simulink model "RF_TX_Model"  (R2026a)
settings: Solver=VariableStepAuto
InitFcn:
  | warning('off')
model workspace (MAT data in the model file):
  Az = 30
  phaseShifts = [20.1529923745; -88.4621483039; 162.922711018; 54.3075703392; -54.3075703392; -162.922711018; 88.4621483039; -20.1529923745]
values from neighbouring files (symbols this model uses):
  BW = 1e8    (= 100000000)    [MatchingNetworkDesign.m]    (also in analyzeReferenceRFBudget.m; build12GHzTransmitterRFBudget.m; build12GHzTransmitterRFBudget_Pin20dBm.m; buildReferenceRFBudgetAnalyzer.m)
  fIF = 4e9    (= 4000000000)    [analyze12GHzTransmitterBudget.m]    (also in analyzeReferenceRFBudget.m; build12GHzTransmitterRFBudget.m; build12GHzTransmitterRFBudget_Pin20dBm.m; buildReferenceRFBudgetAnalyzer.m)
  S = sparameters(rfAntenna,fRF)    [runAntenna2Bits.m]
  splitterCorporate = design(powerDividerCorporate(NumOutputPorts=N,SplitterElement=e), fRF)    [runAntenna2Bits.m]
undefined symbols (not defined in the file or in its folder): rational, sparameters
libraries: simrfV2elements x7, simrfV2_lib x6, dspstat3 x5, simrfV2util1 x3, commrflib2 x1, simrfV2systems x1, simrfV2private x1, dspmathops x1
(part 1 of 3)
settings Model: Creator=gzucchel  LastModifiedBy=gzucchel
settings DataIOCC: SaveFinalState=on  SaveOperatingPoint=on

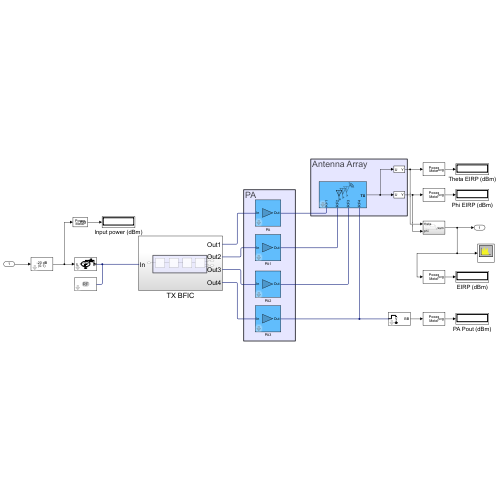
[thumbnail: Simulink's stored preview of the top-level diagram]
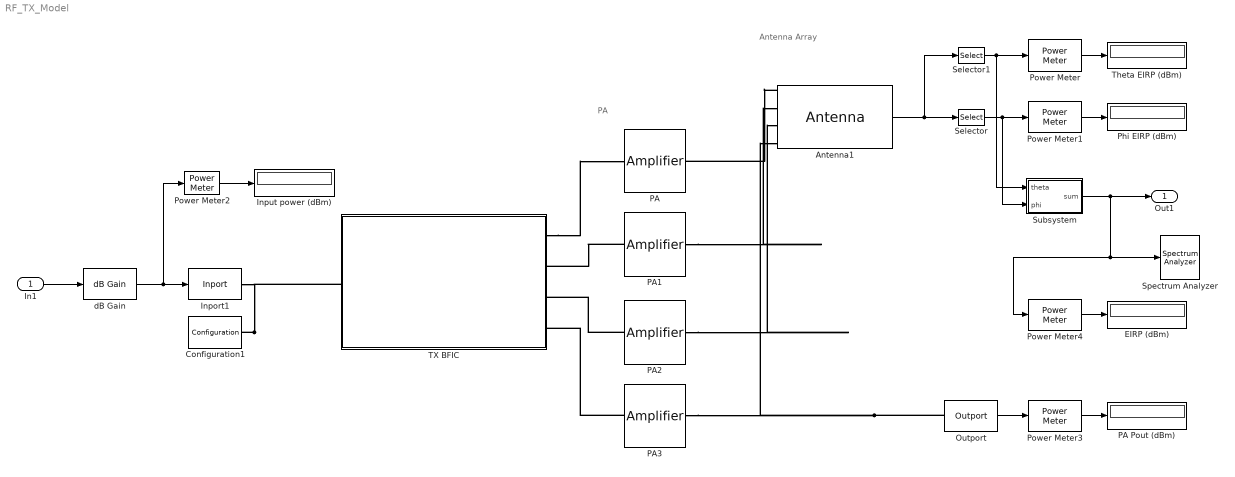
== system RF_TX_Model ==
  note: Antenna Array
  note: PA
  In1 : Inport  PortDimensions=1  SampleTime=2.03450520833333e-09  Interpolate=off
      settings: SignalType=complex
  Antenna1 : simrfV2elements/Antenna  CacheLevel=0  AntennaSource=Antenna object  PrevAppliedAntSource=Antenna object  Gr=0 dBi  Zin=50  AntennaObj=antennaArray  InputIncWave=off  OutputRadWave=on  CarrierFreqInc=2.1 GHz  rArr=[180 0] deg  CarrierFreqRad=12 GHz  rDep=[90 0] deg  AddNoise=off  InternalGrounding=on  SparamRepresentationImp=Frequency domain  FitTolImp=-40  AutoImpulseLengthImp=on  ImpulseLengthImp=1e-10 s
  Configuration1 : simrfV2util1/Configuration  AutoFreq=off  Tones=[4] GHz  Harmonics=3  NormalizeCarrierPower=on  SolverType=Auto  UseCCode=on  StepSize=2.03450520833333e-09 s  AddNoise=on  defaultRNG=on  Seed=0  Temperature=290.0 K  SolverDelFlag=0  AbsTol=1e-6  RelTol=1e-3  MaxIter=10  ErrorEstimationType=2-norm over all variables  EnableInterpFilter=on  HiddenFIRfilterControllerParam=on  SmallSignalApprox=off  AllSimFreqs=on  SimFreqs=[] Hz  SimFreqsInternal=[]  SamplesPerFrame=1
  EIRP (dBm) : Display
  Inport1 : simrfV2util1/Inport  SimulinkInputSignalType=Power  CarrierFreq=[4] GHz  ZS=50  UseSqWave=off  NumCoeff=10  Bias=0  DutyCyc=50  AddNoise=on  InternalGrounding=on
  Input power (dBm) : Display
  Outport : simrfV2util1/Outport  SensorType=Ideal voltage  OutputFormat=Complex Baseband  CarrierFreq=12 GHz  ZL=Inf  AddNoise=off  InternalGrounding=on  StepSize=1e-6 s  AutoStep=on  HalfPolyphaseLength=12
  PA{,1..3} (4 alike) : simrfV2elements/Amplifier  classname=amplifier  DataSource=Data file  File=unitygain.s2p  isNetworkObj=off  NetworkObject=sparameters('default.s2p')  Paramtype=S-parameters  Sparam=[0 0;1 0]  SparamFreq=1e9 Hz  SparamZ0=50  isRationalObj=off  RationalObject=rational('default.s2p')  Residues=0  Poles=0  DF={0 0; 1 0}  Source_linear_gain=Available power gain  linear_gain=25 dB  AmAmAmPmTable=[-25,5,-1;-10,20,-2;0,27,5;5,28,12]  Zin=50  Zout=50  Source_Poly=Odd order  Poly_Coeffs=[0 1]  IPType=Output  IP2=Inf dBm  IP3=45 dBm  P1dB=33 dBm  Psat=36 dBm  Gcomp=inf dBm  InternalGrounding=on  SourceFreq=Extracted from data source  PlotFreq=[1e9:1e6:3e9] Hz  PlotType=X-Y plane  YParam1=S(1,1)  YFormat1=Magnitude (dB)  YParam2=None  YFormat2=Magnitude (dB)  YOption=Linear  XOption=Linear  SparamRepresentation=Time domain  FitTol=-40  FitOpt=Fit individually  MaxPoles=48  AutoImpulseLength=on  ImpulseLength=1e-10 s  MagModeling=off  AddNoise=on  NoiseType=Noise figure  NoiseDist=White  NF=6  MinNF=0  Gopt=0  RN=0  CarrierFreq=0 Hz  NoiseAutoImpulseLength=on  NoiseImpulseLength=1e-10 s  ConstS21NL=off  OpFreq=1 GHz  SetOpFreqAsMaxS21=on
  PA Pout (dBm) : Display
  Phi EIRP (dBm) : Display
  Power Meter{,1..2,4} (4 alike) : dspstat3/Power Meter  Measurement=Average power  ReferenceLoad=1  OutputPowerUnits=dBm  WindowLength=256  OverlapLength=255  AllowArbitraryInputLength=off  ComputeCCDF=off  PowerRange=50  PowerResolution=0.1  CCDFOutput=Relative power (dB above average power)  ProbabilityVector=[ 10; 1; 0.1; 0.01; 0.001; 0.0001 ]  RelativePowerVector=[ 0; 3; 6; 9; 12 ]  ResetPort=off  SimulateUsing=Code generation
      settings: LibrarySourceBlock=commutil2/Power Meter
  Power Meter3 : dspstat3/Power Meter  Measurement=Average power  ReferenceLoad=50  OutputPowerUnits=dBm  WindowLength=256  OverlapLength=255  AllowArbitraryInputLength=off  ComputeCCDF=off  PowerRange=50  PowerResolution=0.1  CCDFOutput=Relative power (dB above average power)  ProbabilityVector=[ 10; 1; 0.1; 0.01; 0.001; 0.0001 ]  RelativePowerVector=[ 0; 3; 6; 9; 12 ]  ResetPort=off  SimulateUsing=Code generation
      settings: LibrarySourceBlock=commutil2/Power Meter
  Selector : Selector  NumberOfDimensions=3  InputPortWidth=3  IndexOptions=Index vector (dialog),Index vector (dialog),Index vector (dialog)  Indices=1,1,2  OutputSizes=1,1,1
  Selector1 : Selector  NumberOfDimensions=3  InputPortWidth=3  IndexOptions=Index vector (dialog),Index vector (dialog),Index vector (dialog)  Indices=1,1,1  OutputSizes=1,1,1
  Spectrum Analyzer : SpectrumAnalyzer  WindowPosition=[55.000000,61.000000,800.000000,500.000000,]  Visible=on  ScopeFrameLocation=window  RBWSource=Property  RBW=1e6  WindowInvariantSamplesPerUpdate=on  Span=491520000  CenterFrequency=8000000000  StartFrequency=7754240000  StopFrequency=8245760000  FrequencyOffset=8000000000  YLimits=[-31.4012 21.4573]  SelectedToolstripTab=spectrumAnalyzerToolstrip.channelMeasurementsTab
  Subsystem : Subsystem
  TX BFIC : Subsystem
  Theta EIRP (dBm) : Display
  dB Gain : dspmathops/dB Gain  dB=Pin  intype=Amplitude
  Out1 : Outport  PortDimensions=1  SampleTime=2.03450520833333e-09
  wires:
  In1/1 -> dB Gain/1
  Power Meter1/1 -> Phi EIRP (dBm)/1
  Power Meter2/1 -> Input power (dBm)/1
  dB Gain/1 -> Inport1/1, Power Meter2/1
  Selector/1 -> Subsystem/2(phi), Power Meter1/1
  Selector1/1 -> Power Meter/1, Subsystem/1(theta)
  Antenna1/1 -> Selector1/1, Selector/1
  Power Meter/1 -> Theta EIRP (dBm)/1
  Power Meter3/1 -> PA Pout (dBm)/1
  Outport/1 -> Power Meter3/1
  Subsystem/1(sum) -> Power Meter4/1, Spectrum Analyzer/1, Out1/1
  Power Meter4/1 -> EIRP (dBm)/1
  connections:
  PA2/RConn1 -- Antenna1/LConn3
  Antenna1/LConn1 -- PA/RConn1
  PA1/RConn1 -- Antenna1/LConn2
  PA3/RConn1 -- Outport/LConn1 -- Antenna1/LConn4
  Configuration1/LConn1 -- TX BFIC/LConn1 -- Inport1/RConn1
  TX BFIC/RConn1 -- PA/LConn1
  PA1/LConn1 -- TX BFIC/RConn2
  PA2/LConn1 -- TX BFIC/RConn3
  PA3/LConn1 -- TX BFIC/RConn4

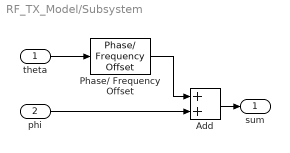
== system RF_TX_Model/Subsystem ==
  theta : Inport
  phi : Inport  Port=2
  Add : Sum
  Phase/ Frequency Offset : commrflib2/Phase// Frequency Offset  PhaseOffset=-90  FrequencyOffsetFromPort=off  FrequencyOffset=0  SimulateUsing=Code generation
  sum : Outport
  wires:
  phi/1 -> Add/2
  Add/1 -> sum/1
  theta/1 -> Phase/ Frequency Offset/1
  Phase/ Frequency Offset/1 -> Add/1

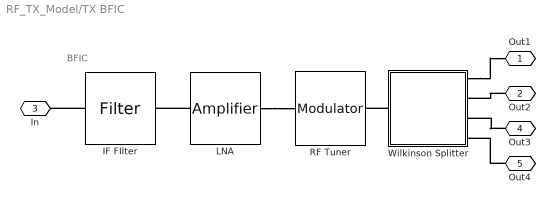
== system RF_TX_Model/TX BFIC ==
  note: BFIC
  IF FIlter : simrfV2elements/Filter  classname=filter  DesignMethod=InverseChebyshev  ResponseType=Bandpass  Implementation=LC Tee  ImplementationIdeal=Constant per carrier  ImplementationRational=Transfer function  UseFilterOrder=on  FilterOrder=5  PassFreq_lp=1 GHz  PassFreq_hp=2 GHz  PassFreq_bp=[-BW/2 BW/2]+fIF Hz  PassFreq_bs=[1 4] GHz  PassAtten=3  StopFreq_lp=2 GHz  StopFreq_hp=1 GHz  StopFreq_bp=[1.5 3.5] GHz  StopFreq_bs=[2.1 2.9] GHz  StopAtten=40  Rsrc=50  Rload=50  AutoImpulseLength=on  ImpulseLength=1e-10 s  InternalGrounding=on  PlotFuncLeft=Voltage transfer  PlotLeftForm=Magnitude (dB)  PlotRightOnVT=None  PlotRightNoTD=None  PlotRightNoGD=None  PlotRightNoIR=None  PlotRightNoSR=None  PlotRightForm=Magnitude (dB)  FreqPoints=logspace(0,10,101)  Freq_unit=Hz  TimePoints=linspace(0,1,1e6+1)  Time_unit=s  XaxisScale=Linear  YaxisScale=Linear  needRedraw=1
  LNA : simrfV2elements/Amplifier  classname=amplifier  DataSource=Data file  File=CMD240withNF.s2p  isNetworkObj=off  NetworkObject=sparameters('default.s2p')  Paramtype=S-parameters  Sparam=[0 0;1 0]  SparamFreq=1e9 Hz  SparamZ0=50  isRationalObj=off  RationalObject=rational('default.s2p')  Residues=0  Poles=0  DF={0 0; 1 0}  Source_linear_gain=Data source  linear_gain=0 dB  AmAmAmPmTable=[-25,5,-1;-10,20,-2;0,27,5;5,28,12]  Zin=50  Zout=50  Source_Poly=Even and odd order  Poly_Coeffs=[0 1]  IPType=Output  IP2=Inf dBm  IP3=28 dBm  P1dB=inf dBm  Psat=inf dBm  Gcomp=inf dBm  InternalGrounding=on  SourceFreq=Extracted from data source  PlotFreq=[1e9:1e6:3e9] Hz  PlotType=X-Y plane  YParam1=S(2,1)  YFormat1=Magnitude (dB)  YParam2=None  YFormat2=Magnitude (dB)  YOption=Linear  XOption=Linear  SparamRepresentation=Time domain  FitTol=-30  FitOpt=Fit individually  MaxPoles=48  AutoImpulseLength=on  ImpulseLength=1e-10 s  MagModeling=off  AddNoise=on  NoiseType=Noise figure  NoiseDist=White  NF=0  MinNF=0  Gopt=0  RN=0  CarrierFreq=0 Hz  NoiseAutoImpulseLength=on  NoiseImpulseLength=1e-10 s  ConstS21NL=off  OpFreq=4 GHz  SetOpFreqAsMaxS21=on
  RF Tuner : simrfV2systems/Modulator  classname=rfmod  Source_linear_gain=Available power gain  linear_gain=6 dB  Poly_Coeffs=[0 1]  LOFreq=8 GHz  Zin=50  Zout=50  AddIRFilter=off  AddCSFilter=off  InternalGrounding=on  ForceNextInit=off  Source_Poly=Even and odd order  IPType=Output  IP2=Inf dBm  IP3=32 dBm  P1dB=inf dBm  Psat=inf dBm  Gcomp=inf dBm  NF=3  Isolation=inf dB  AddPhaseNoise=off  PhaseNoiseOffset=1  PhaseNoiseLevel=-Inf  AutoImpulseLengthPN=on  ImpulseLengthPN=1e-10  ImpulseLength_unitPN=s  DesignMethodIR=Ideal  ResponseTypeIR=Lowpass  ImplementationIR=LC Tee  ImplementationIdealIR=Constant per carrier  ImplementationRationalIR=Transfer function  UseFilterOrderIR=on  FilterOrderIR=3  PassFreq_lpIR=4.05  PassFreq_lp_unitIR=GHz  PassFreq_hpIR=3.95  PassFreq_hp_unitIR=GHz  PassFreq_bpIR=[3.95 4.05]  PassFreq_bp_unitIR=GHz  PassFreq_bsIR=[49.949999999 50.050000001]  PassFreq_bs_unitIR=GHz  PassAttenIR=10*log10(2)  StopFreq_lpIR=4.050000001  StopFreq_lp_unitIR=GHz  StopFreq_hpIR=3.949999999  StopFreq_hp_unitIR=GHz  StopFreq_bpIR=[3.949999999 4.050000001]  StopFreq_bp_unitIR=GHz  StopFreq_bsIR=[49.95 50.05]  StopFreq_bs_unitIR=GHz  StopAttenIR=40  RsrcIR=50  RloadIR=50  AutoImpulseLengthIR=on  ImpulseLengthIR=1e-10  ImpulseLength_unitIR=s  DesignMethodCS=Ideal  ResponseTypeCS=Highpass  ImplementationCS=LC Tee  ImplementationIdealCS=Constant per carrier  ImplementationRationalCS=Transfer function  UseFilterOrderCS=on  FilterOrderCS=3  PassFreq_lpCS=27.05  PassFreq_lp_unitCS=GHz  PassFreq_hpCS=26.95  PassFreq_hp_unitCS=GHz  PassFreq_bpCS=[26.95 27.05]  PassFreq_bp_unitCS=GHz  PassFreq_bsCS=[18.949999999 19.050000001]  PassFreq_bs_unitCS=GHz  PassAttenCS=10*log10(2)  StopFreq_lpCS=27.050000001  StopFreq_lp_unitCS=GHz  StopFreq_hpCS=26.949999999  StopFreq_hp_unitCS=GHz  StopFreq_bpCS=[26.949999999 27.050000001]  StopFreq_bp_unitCS=GHz  StopFreq_bsCS=[18.95 19.05]  StopFreq_bs_unitCS=GHz  StopAttenCS=40  RsrcCS=50  RloadCS=50  AutoImpulseLengthCS=on  ImpulseLengthCS=1e-10  ImpulseLength_unitCS=s
  Wilkinson Splitter : Subsystem  DialogController=simrfV2DDGCreate  mask(PCB Block){classname=rfpcb, component=pcb, ObjectPCB=splitterCorporate, AddNoise=on, InternalGrounding=on, SparamRepresentation=Time domain, FitOpt=Share all poles, FitTol=-40, MaxPoles=48, AutoImpulseLength=on, ImpulseLength=1e-10, ImpulseLength_unit=s, SourceFreq=Extracted from data source, PlotFreq=[1e9:1e6:3e9], PlotFreq_unit=Hz, PlotType=X-Y plane, YParam1=S(2,1), YFormat1=Magnitude (dB), YParam2=S(1,1), YFormat2=Magnitude (dB), YOption=Linear, XOption=Linear}
      mask prompts: classname "Class name:"; ObjectPCB "Object:"; AddNoise "Simulate noise"; InternalGrounding "Ground and hide negative terminals."; SparamRepresentation "S-parameter modeling"; FitOpt "S-parameters fitting:"; FitTol "Fit tolerance (dB):"; MaxPoles "Maximum number of poles:"; AutoImpulseLength "Automatically estimate impulse response duration"; ImpulseLength "Impulse response duration:"; ImpulseLength_unit "Impulse response duration unit:"; SourceFreq "Source of frequency data:"; PlotFreq "Frequency range for plotting:"; PlotFreq_unit "Plot frequency unit:"; PlotType "Plot type:"; YParam1 "Plot parameter1:"; YFormat1 "Plot format1:"; YParam2 "Plot parameter2:"; YFormat2 "Plot format2:"; YOption "Y option:"; XOption "X option:"
      mask help: Model an PCB component.
      mask init:
      | simrfV2rfpcb(gcb,'simrfInit');
      settings: CopyFcn=simrfV2rfpcb(gcb, 'simrfCopy');
      mask Help: eval('simrfV2_help(gcbh)')
      mask TypeOptions SparamRepresentation: Time domain | Frequency domain
      mask TypeOptions FitOpt: Share poles by columns | Share all poles | Fit individually
      mask TypeOptions ImpulseLength_unit: s | ms | us | ns | ps
      mask TypeOptions SourceFreq: User-specified | Extracted from data source
      mask TypeOptions PlotFreq_unit: Hz | kHz | MHz | GHz
      mask TypeOptions PlotType: X-Y plane | Polar plane | Z Smith chart | Y Smith chart | ZY Smith chart
      mask TypeOptions YParam1: S(1,1) | S(1,2) | S(1,3) | S(1,4) | S(1,5) | S(2,1) | S(2,2) | S(2,3) | S(2,4) | S(2,5) | S(3,1) | S(3,2) | S(3,3) | S(3,4) | S(3,5) | S(4,1) | S(4,2) | S(4,3) | S(4,4) | S(4,5) | S(5,1) | S(5,2) | S(5,3) | S(5,4) | S(5,5)
      mask TypeOptions YFormat1: Magnitude (dB) | Magnitude (linear) | Angle (degrees) | Real | Imaginary
      mask TypeOptions YParam2: None | S(1,1) | S(1,2) | S(1,3) | S(1,4) | S(1,5) | S(2,1) | S(2,2) | S(2,3) | S(2,4) | S(2,5) | S(3,1) | S(3,2) | S(3,3) | S(3,4) | S(3,5) | S(4,1) | S(4,2) | S(4,3) | S(4,4) | S(4,5) | S(5,1) | S(5,2) | S(5,3) | S(5,4) | S(5,5)
      mask TypeOptions YFormat2: Magnitude (dB) | Magnitude (linear) | Angle (degrees) | Real | Imaginary
      mask TypeOptions YOption: Linear | Logarithmic
      mask TypeOptions XOption: Linear | Logarithmic
      mask Display:
      | port_label('LConn', 1,'1')
      | port_label('RConn', 1,'2')
      | port_label('RConn', 2,'3')
      | port_label('RConn', 3,'4')
      | port_label('RConn', 4,'5')
  Out1 : PMIOPort  Side=Right
  Out2 : PMIOPort  Port=2  Side=Right
  In : PMIOPort  Port=3  Side=Left
  Out3 : PMIOPort  Port=4  Side=Right
  Out4 : PMIOPort  Port=5  Side=Right
  connections:
  LNA/LConn1 -- IF FIlter/RConn1
  Wilkinson Splitter/LConn1 -- RF Tuner/RConn1
  LNA/RConn1 -- RF Tuner/LConn1
  Out2/RConn1 -- Wilkinson Splitter/RConn2
  Wilkinson Splitter/RConn1 -- Out1/RConn1
  Out3/RConn1 -- Wilkinson Splitter/RConn3
  IF FIlter/LConn1 -- In/RConn1
  Out4/RConn1 -- Wilkinson Splitter/RConn4
